simulink model "mfordmodel_v1"  (R2023a)
settings: Solver=ode45  StartTime=0.0  StopTime=10.0  RelTol=1e-3  EnableMultiTasking=on
undefined symbols (not defined in the file): ABV_RATIO_SW, AC_OFF_DLY, ACLOD, AUTO_TRNS_SW, BRAKE_DNDT_X, BZZRPM, BZZRPM_ALT, BZZTM, BZZTM_ALT, CMD_LITOFF, CMD_STABLE, CO_ST_ECT__A, COOL_BASE, DAS_BKDLY_A, DAS_CNT, DAS_CTDLY, DAS_LC_SW__A, DASCLP_5INH, DASCTL, DASMHYST, DASMPH, DEBYCP, DES_BASE, DPNEU_MUL, DSDRPM_DN_TC, DSDRPM_OFF, DSDRPM_UP_TC, EDF_DELAY, EDFHP, ETC_CL_TP, ETC_HP, GR_CM_CREEP, HCAM_ACT_CLP, HEDFHP, HEDFRPM, HICAM_PS, IAC_CAL_SW, IAC_ER_TM1, IAC_ER_TM2, IAC_ER_TM4, IAC_HI_LIM__A, IAC_ISFL_OBD, IAC_KAM_SW, IAC_LO_LIM__A, IAC_MON_TM, IAC_OT_REQ, IAC_RUN_TM, IAC_TP_OBD, IAC_TR_DAS, IAC_TST_DC, ID_DAS__A, ID_NOVS__A, IDVS_CH__A, IDVS_SL__A, IPSI_SW, IPSIDLY, IS_DRBASE__A, IS_DRBASE_A__A, IS_NUBASE__A, IS_NUBASE_A__A ... (+35)
libraries: simulink x2
(part 9 of 12)

== system mfordmodel_v1/iac_v04_001_001/normal_mode/iscflg_module/dashpot/TIMER/Time Calculator ==
  note: Calculates timer value.
      | Activated only when
      | counting up or down.
  note: Calculates time
      | between cycles.
      | Activated every cycle.
  note: Resets timer
      | to 'reset_value'
  note: Increment, hold,
      | or decrement
  note: Timer Control calls the counters 'delta_time' and 'timer_calculation'
      | after using the flags 'increment_flag' and 'decrement_flag'
      | to determine the direction of the timer.
  note: timer14/TIMER/Time Calculator
  count_direction : Inport
  reset_val : Inport  Port=2
  do_delta_time : Inport  Port=3
  do_timer : Inport  Port=4
  reset_value : Inport  Port=5
  From : From
  Goto : Goto
  delta_time : Subsystem  TreatAsAtomicUnit=on
  timer_calculation : Subsystem  TreatAsAtomicUnit=on
  timer : Outport
  wires:
  reset_value/1 -> timer_calculation/1(reset_value)  "reset_value"
  reset_val/1 -> timer_calculation/2(reset_flag)  "reset_flag"
  do_timer/1 -> timer_calculation/Trigger  "do_timer"
  From/1 -> timer_calculation/3(delta_time)  "delta_time"
  timer_calculation/1(timer) -> timer/1  "timer"
  count_direction/1 -> delta_time/1(count_direction)  "count_direction"
  delta_time/1(delta_time) -> Goto/1  "delta_time"
  do_delta_time/1 -> delta_time/Trigger  "do_delta_time"

== system mfordmodel_v1/iac_v04_001_001/normal_mode/iscflg_module/dashpot/daspot_calc/ROLAV_TC_in_DT_in ==
  note: Using the first two terms of the series expansion:
      |
      |                     x                     x2
      |                                e   =  1  +  x  +  --  + ......
      |                                           2!
      |
      |       Simplifying, the exponential "f" becomes:
      |
      |                  - (FK_TMR/TC)              1
      |           f  =  1  -  e                    =  1  -  -------------  =  . . .
      |                                                    (FK_TMR/TC)
      |                           e
      |
      |                              1                      1
      |          f  =  1  -  ---------------------------------  =    ------------------- .
      |                                  1 + (FK_TMR / TC)       1 + (TC / FK_TMR)
  note: - (FK_TMR/TC)
      |                                    f  =  1  -  e
      |
      |       Where "f" is called the filter constant in the difference equation:
      |
      |                    new_average = f * new_value + (1 - f) * old_average
  note: new_average = [ (sample_interval)/(sample_interval + time_constant) ] * (new_value - old_ave) + old_ave
  new_value : Inport
  Tau : Inport  Port=2
  old_ave : Inport  Port=3
  delta_time : Inport  Port=4
  Elementary Math : Math  Operator=reciprocal  SignedPower=on
  Product : Product  Inputs=3  InputSameDT=on  RndMeth=Zero  SaturateOnIntegerOverflow=on  OutDataTypeStr=Inherit: Same as first input
  Sum : Sum  Inputs=-+  InputSameDT=on  SaturateOnIntegerOverflow=on  OutDataTypeStr=Inherit: Same as first input
  Sum1 : Sum  InputSameDT=on  SaturateOnIntegerOverflow=on  OutDataTypeStr=Inherit: Same as first input
  Sum2 : Sum  InputSameDT=on  SaturateOnIntegerOverflow=on  OutDataTypeStr=Inherit: Same as first input
  new_ave : Outport
  wires:
  delta_time/1 -> Product/2, Sum1/1
  Tau/1 -> Sum1/2
  Sum2/1 -> new_ave/1
  old_ave/1 -> Sum2/1, Sum/1
  Product/1 -> Sum2/2
  Sum/1 -> Product/1
  Elementary Math/1 -> Product/3
  Sum1/1 -> Elementary Math/1
  new_value/1 -> Sum/2

== system mfordmodel_v1/iac_v04_001_001/normal_mode/iscflg_module/dashpot/daspot_calc/lookup_2d ==
  In1 : Inport
  Look-Up Table1 : Lookup  InputValues=calfunc.X  Table=calfunc.Y
  Saturation1 : Saturate  UpperLimit=max_x  LowerLimit=min_x
  Out1 : Outport
  wires:
  In1/1 -> Saturation1/1
  Saturation1/1 -> Look-Up Table1/1
  Look-Up Table1/1 -> Out1/1

== system mfordmodel_v1/iac_v04_001_001/normal_mode/iscflg_module/dashpot/daspot_calc/lookup_2d2 ==
  In1 : Inport
  Look-Up Table1 : Lookup  InputValues=calfunc.X  Table=calfunc.Y
  Saturation1 : Saturate  UpperLimit=max_x  LowerLimit=min_x
  Out1 : Outport
  wires:
  In1/1 -> Saturation1/1
  Saturation1/1 -> Look-Up Table1/1
  Look-Up Table1/1 -> Out1/1

== system mfordmodel_v1/iac_v04_001_001/normal_mode/iscflg_module/dashpot/function_calcs/lookup_2d ==
  In1 : Inport
  Look-Up Table1 : Lookup  InputValues=calfunc.X  Table=calfunc.Y
  Saturation1 : Saturate  UpperLimit=max_x  LowerLimit=min_x
  Out1 : Outport
  wires:
  In1/1 -> Saturation1/1
  Saturation1/1 -> Look-Up Table1/1
  Look-Up Table1/1 -> Out1/1

== system mfordmodel_v1/iac_v04_001_001/normal_mode/iscflg_module/dashpot/function_calcs/lookup_2d1 ==
  In1 : Inport
  Look-Up Table1 : Lookup  InputValues=calfunc.X  Table=calfunc.Y
  Saturation1 : Saturate  UpperLimit=max_x  LowerLimit=min_x
  Out1 : Outport
  wires:
  In1/1 -> Saturation1/1
  Saturation1/1 -> Look-Up Table1/1
  Look-Up Table1/1 -> Out1/1

== system mfordmodel_v1/iac_v04_001_001/normal_mode/iscflg_module/dashpot/function_calcs/lookup_2d2 ==
  In1 : Inport
  Look-Up Table1 : Lookup  InputValues=calfunc.X  Table=calfunc.Y
  Saturation1 : Saturate  UpperLimit=max_x  LowerLimit=min_x
  Out1 : Outport
  wires:
  In1/1 -> Saturation1/1
  Saturation1/1 -> Look-Up Table1/1
  Look-Up Table1/1 -> Out1/1

== system mfordmodel_v1/iac_v04_001_001/normal_mode/iscflg_module/dashpot/function_calcs/lookup_2d3 ==
  In1 : Inport
  Look-Up Table1 : Lookup  InputValues=calfunc.X  Table=calfunc.Y
  Saturation1 : Saturate  UpperLimit=max_x  LowerLimit=min_x
  Out1 : Outport
  wires:
  In1/1 -> Saturation1/1
  Saturation1/1 -> Look-Up Table1/1
  Look-Up Table1/1 -> Out1/1

== system mfordmodel_v1/iac_v04_001_001/normal_mode/iscflg_module/dashpot/function_calcs/lookup_2d4 ==
  In1 : Inport
  Look-Up Table1 : Lookup  InputValues=calfunc.X  Table=calfunc.Y
  Saturation1 : Saturate  UpperLimit=max_x  LowerLimit=min_x
  Out1 : Outport
  wires:
  In1/1 -> Saturation1/1
  Saturation1/1 -> Look-Up Table1/1
  Look-Up Table1/1 -> Out1/1

== system mfordmodel_v1/iac_v04_001_001/normal_mode/iscflg_module/dashpot/function_calcs/lookup_2d5 ==
  In1 : Inport
  Look-Up Table1 : Lookup  InputValues=calfunc.X  Table=calfunc.Y
  Saturation1 : Saturate  UpperLimit=max_x  LowerLimit=min_x
  Out1 : Outport
  wires:
  In1/1 -> Saturation1/1
  Saturation1/1 -> Look-Up Table1/1
  Look-Up Table1/1 -> Out1/1

== system mfordmodel_v1/iac_v04_001_001/normal_mode/iscflg_module/dashpot/function_calcs/lookup_2d6 ==
  In1 : Inport
  Look-Up Table1 : Lookup  InputValues=calfunc.X  Table=calfunc.Y
  Saturation1 : Saturate  UpperLimit=max_x  LowerLimit=min_x
  Out1 : Outport
  wires:
  In1/1 -> Saturation1/1
  Saturation1/1 -> Look-Up Table1/1
  Look-Up Table1/1 -> Out1/1

== system mfordmodel_v1/iac_v04_001_001/normal_mode/iscflg_module/dashpot/function_calcs/lookup_2d7 ==
  In1 : Inport
  Look-Up Table1 : Lookup  InputValues=calfunc.X  Table=calfunc.Y
  Saturation1 : Saturate  UpperLimit=max_x  LowerLimit=min_x
  Out1 : Outport
  wires:
  In1/1 -> Saturation1/1
  Saturation1/1 -> Look-Up Table1/1
  Look-Up Table1/1 -> Out1/1

== system mfordmodel_v1/iac_v04_001_001/normal_mode/iscflg_module/idle_drive_rpm_controller/idle_ppm_calc/ 1 ==
  In1 : Inport
  Look-Up Table1 : Lookup  InputValues=calfunc.X  Table=calfunc.Y
  Saturation1 : Saturate  UpperLimit=max_x  LowerLimit=min_x
  Out1 : Outport
  wires:
  In1/1 -> Saturation1/1
  Saturation1/1 -> Look-Up Table1/1
  Look-Up Table1/1 -> Out1/1

== system mfordmodel_v1/iac_v04_001_001/normal_mode/iscflg_module/idle_drive_rpm_controller/idle_ppm_calc/CONSTANT7 ==
  Constant : Constant  Value=const
  Out : Outport
  wires:
  Constant/1 -> Out/1

== system mfordmodel_v1/iac_v04_001_001/normal_mode/iscflg_module/idle_drive_rpm_controller/idle_ppm_calc/CONSTANT8 ==
  Constant : Constant  Value=const
  Out : Outport
  wires:
  Constant/1 -> Out/1

== system mfordmodel_v1/iac_v04_001_001/normal_mode/iscflg_module/idle_drive_rpm_controller/idle_ppm_calc/CONSTANT9 ==
  Constant : Constant  Value=const
  Out : Outport
  wires:
  Constant/1 -> Out/1

== system mfordmodel_v1/iac_v04_001_001/normal_mode/iscflg_module/idle_drive_rpm_controller/idle_ppm_calc/VAR_SATURATION1 ==
  note: IF INPUT <= MIN THEN SWITCH MIN ON
  note: IF INPUT >= MAX THEN SWITHMAX ON
  MAX : Inport
  INPUT : Inport  Port=2
  MIN : Inport  Port=3
  From : From
  From1 : From
  Goto : Goto
  Logical Operator : Logic  Operator=OR
  Relational Operator : RelationalOperator
  Relational Operator1 : RelationalOperator  Operator=<=
  Switch : Switch  Threshold=0.5
  Switch2 : Switch  Threshold=0.5
  SwitchMAX : Switch  Threshold=0.5
  OUTPUT : Outport
  LIMIT_FLAG : Outport  Port=2
  wires:
  MIN/1 -> Switch/1, Relational Operator1/2
  Switch/1 -> Switch2/3
  From1/1 -> SwitchMAX/3
  From/1 -> Switch/3
  INPUT/1 -> Goto/1, Relational Operator1/1, Relational Operator/1
  Switch2/1 -> OUTPUT/1
  SwitchMAX/1 -> Switch2/1
  MAX/1 -> SwitchMAX/1, Relational Operator/2
  Relational Operator/1 -> SwitchMAX/2, Switch2/2, Logical Operator/1
  Relational Operator1/1 -> Switch/2, Logical Operator/2
  Logical Operator/1 -> LIMIT_FLAG/1

== system mfordmodel_v1/iac_v04_001_001/normal_mode/iscflg_module/idle_drive_rpm_controller/idle_ppm_calc/VAR_SATURATION2 ==
  note: IF INPUT <= MIN THEN SWITCH MIN ON
  note: IF INPUT >= MAX THEN SWITHMAX ON
  MAX : Inport
  INPUT : Inport  Port=2
  MIN : Inport  Port=3
  From : From
  From1 : From
  Goto : Goto
  Logical Operator : Logic  Operator=OR
  Relational Operator : RelationalOperator
  Relational Operator1 : RelationalOperator  Operator=<=
  Switch : Switch  Threshold=0.5
  Switch2 : Switch  Threshold=0.5
  SwitchMAX : Switch  Threshold=0.5
  OUTPUT : Outport
  LIMIT_FLAG : Outport  Port=2
  wires:
  MIN/1 -> Switch/1, Relational Operator1/2
  Switch/1 -> Switch2/3
  From1/1 -> SwitchMAX/3
  From/1 -> Switch/3
  INPUT/1 -> Goto/1, Relational Operator1/1, Relational Operator/1
  Switch2/1 -> OUTPUT/1
  SwitchMAX/1 -> Switch2/1
  MAX/1 -> SwitchMAX/1, Relational Operator/2
  Relational Operator/1 -> SwitchMAX/2, Switch2/2, Logical Operator/1
  Relational Operator1/1 -> Switch/2, Logical Operator/2
  Logical Operator/1 -> LIMIT_FLAG/1

== system mfordmodel_v1/iac_v04_001_001/normal_mode/iscflg_module/idle_drive_rpm_controller/idnerr_fil_calc/CONSTANT1 ==
  Constant : Constant  Value=const
  Out : Outport
  wires:
  Constant/1 -> Out/1

== system mfordmodel_v1/iac_v04_001_001/normal_mode/iscflg_module/idle_drive_rpm_controller/idnerr_fil_calc/ROLAV_TC_DT_in1 ==
  note: Using the first two terms of the series expansion:
      |
      |                     x                     x2
      |                                e   =  1  +  x  +  --  + ......
      |                                           2!
      |
      |       Simplifying, the exponential "f" becomes:
      |
      |                  - (FK_TMR/TC)              1
      |           f  =  1  -  e                    =  1  -  -------------  =  . . .
      |                                                    (FK_TMR/TC)
      |                           e
      |
      |                              1                      1
      |          f  =  1  -  ---------------------------------  =    ------------------- .
      |                                  1 + (FK_TMR / TC)       1 + (TC / FK_TMR)
  note: - (FK_TMR/TC)
      |                                    f  =  1  -  e
      |
      |       Where "f" is called the filter constant in the difference equation:
      |
      |                    new_average = f * new_value + (1 - f) * old_average
  note: new_average = [ (sample_interval)/(sample_interval + time_constant) ] * (new_value - old_ave) + old_ave
  new_value : Inport
  old_ave : Inport  Port=2
  delta_time : Inport  Port=3
  Elementary Math : Math  Operator=reciprocal  SignedPower=on
  Product : Product  Inputs=3  InputSameDT=on  RndMeth=Zero  SaturateOnIntegerOverflow=on  OutDataTypeStr=Inherit: Same as first input
  Sum : Sum  Inputs=-+  InputSameDT=on  SaturateOnIntegerOverflow=on  OutDataTypeStr=Inherit: Same as first input
  Sum1 : Sum  InputSameDT=on  SaturateOnIntegerOverflow=on  OutDataTypeStr=Inherit: Same as first input
  Sum2 : Sum  InputSameDT=on  SaturateOnIntegerOverflow=on  OutDataTypeStr=Inherit: Same as first input
  Time Constant : Constant  Value=tc
  new_ave : Outport
  wires:
  Time Constant/1 -> Sum1/2
  Sum2/1 -> new_ave/1
  old_ave/1 -> Sum2/1, Sum/1
  Product/1 -> Sum2/2
  Sum/1 -> Product/1
  Elementary Math/1 -> Product/3
  Sum1/1 -> Elementary Math/1
  new_value/1 -> Sum/2
  delta_time/1 -> Product/2, Sum1/1

== system mfordmodel_v1/iac_v04_001_001/normal_mode/iscflg_module/idle_rpm_controller/fn852a_calc/FN852A ==
  In1 : Inport
  Look-Up Table1 : Lookup  InputValues=calfunc.X  Table=calfunc.Y
  Saturation1 : Saturate  UpperLimit=max_x  LowerLimit=min_x
  Out1 : Outport
  wires:
  In1/1 -> Saturation1/1
  Saturation1/1 -> Look-Up Table1/1
  Look-Up Table1/1 -> Out1/1

== system mfordmodel_v1/iac_v04_001_001/normal_mode/iscflg_module/idle_rpm_controller/idle_ppm_calc/FN851A ==
  In1 : Inport
  Look-Up Table1 : Lookup  InputValues=calfunc.X  Table=calfunc.Y
  Saturation1 : Saturate  UpperLimit=max_x  LowerLimit=min_x
  Out1 : Outport
  wires:
  In1/1 -> Saturation1/1
  Saturation1/1 -> Look-Up Table1/1
  Look-Up Table1/1 -> Out1/1

== system mfordmodel_v1/iac_v04_001_001/normal_mode/iscflg_module/idle_rpm_controller/idle_ppm_calc/PID_DELTA ==
  Constant : Constant  Value=const
  Out : Outport
  wires:
  Constant/1 -> Out/1

== system mfordmodel_v1/iac_v04_001_001/normal_mode/iscflg_module/idle_rpm_controller/idle_ppm_calc/ROLAV_TC_in_DT_in ==
  note: Using the first two terms of the series expansion:
      |
      |                     x                     x2
      |                                e   =  1  +  x  +  --  + ......
      |                                           2!
      |
      |       Simplifying, the exponential "f" becomes:
      |
      |                  - (FK_TMR/TC)              1
      |           f  =  1  -  e                    =  1  -  -------------  =  . . .
      |                                                    (FK_TMR/TC)
      |                           e
      |
      |                              1                      1
      |          f  =  1  -  ---------------------------------  =    ------------------- .
      |                                  1 + (FK_TMR / TC)       1 + (TC / FK_TMR)
  note: - (FK_TMR/TC)
      |                                    f  =  1  -  e
      |
      |       Where "f" is called the filter constant in the difference equation:
      |
      |                    new_average = f * new_value + (1 - f) * old_average
  note: new_average = [ (sample_interval)/(sample_interval + time_constant) ] * (new_value - old_ave) + old_ave
  new_value : Inport
  Tau : Inport  Port=2
  old_ave : Inport  Port=3
  delta_time : Inport  Port=4
  Elementary Math : Math  Operator=reciprocal  SignedPower=on
  Product : Product  Inputs=3  InputSameDT=on  RndMeth=Zero  SaturateOnIntegerOverflow=on  OutDataTypeStr=Inherit: Same as first input
  Sum : Sum  Inputs=-+  InputSameDT=on  SaturateOnIntegerOverflow=on  OutDataTypeStr=Inherit: Same as first input
  Sum1 : Sum  InputSameDT=on  SaturateOnIntegerOverflow=on  OutDataTypeStr=Inherit: Same as first input
  Sum2 : Sum  InputSameDT=on  SaturateOnIntegerOverflow=on  OutDataTypeStr=Inherit: Same as first input
  new_ave : Outport
  wires:
  delta_time/1 -> Product/2, Sum1/1
  Tau/1 -> Sum1/2
  Sum2/1 -> new_ave/1
  old_ave/1 -> Sum2/1, Sum/1
  Product/1 -> Sum2/2
  Sum/1 -> Product/1
  Elementary Math/1 -> Product/3
  Sum1/1 -> Elementary Math/1
  new_value/1 -> Sum/2

== system mfordmodel_v1/iac_v04_001_001/normal_mode/iscflg_module/idle_rpm_controller/idle_ppm_calc/ROLAV_TC_in_DT_in1 ==
  note: Using the first two terms of the series expansion:
      |
      |                     x                     x2
      |                                e   =  1  +  x  +  --  + ......
      |                                           2!
      |
      |       Simplifying, the exponential "f" becomes:
      |
      |                  - (FK_TMR/TC)              1
      |           f  =  1  -  e                    =  1  -  -------------  =  . . .
      |                                                    (FK_TMR/TC)
      |                           e
      |
      |                              1                      1
      |          f  =  1  -  ---------------------------------  =    ------------------- .
      |                                  1 + (FK_TMR / TC)       1 + (TC / FK_TMR)
  note: - (FK_TMR/TC)
      |                                    f  =  1  -  e
      |
      |       Where "f" is called the filter constant in the difference equation:
      |
      |                    new_average = f * new_value + (1 - f) * old_average
  note: new_average = [ (sample_interval)/(sample_interval + time_constant) ] * (new_value - old_ave) + old_ave
  new_value : Inport
  Tau : Inport  Port=2
  old_ave : Inport  Port=3
  delta_time : Inport  Port=4
  Elementary Math : Math  Operator=reciprocal  SignedPower=on
  Product : Product  Inputs=3  InputSameDT=on  RndMeth=Zero  SaturateOnIntegerOverflow=on  OutDataTypeStr=Inherit: Same as first input
  Sum : Sum  Inputs=-+  InputSameDT=on  SaturateOnIntegerOverflow=on  OutDataTypeStr=Inherit: Same as first input
  Sum1 : Sum  InputSameDT=on  SaturateOnIntegerOverflow=on  OutDataTypeStr=Inherit: Same as first input
  Sum2 : Sum  InputSameDT=on  SaturateOnIntegerOverflow=on  OutDataTypeStr=Inherit: Same as first input
  new_ave : Outport
  wires:
  delta_time/1 -> Product/2, Sum1/1
  Tau/1 -> Sum1/2
  Sum2/1 -> new_ave/1
  old_ave/1 -> Sum2/1, Sum/1
  Product/1 -> Sum2/2
  Sum/1 -> Product/1
  Elementary Math/1 -> Product/3
  Sum1/1 -> Elementary Math/1
  new_value/1 -> Sum/2

== system mfordmodel_v1/iac_v04_001_001/normal_mode/iscflg_module/idle_rpm_controller/idle_ppm_calc/TCBPA_DER ==
  Constant : Constant  Value=const
  Out : Outport
  wires:
  Constant/1 -> Out/1

== system mfordmodel_v1/iac_v04_001_001/normal_mode/iscflg_module/idle_rpm_controller/idle_ppm_calc/TCPRO_GT ==
  Constant : Constant  Value=const
  Out : Outport
  wires:
  Constant/1 -> Out/1

== system mfordmodel_v1/iac_v04_001_001/normal_mode/iscflg_module/idle_rpm_controller/idle_ppm_calc/TCPRO_LT ==
  Constant : Constant  Value=const
  Out : Outport
  wires:
  Constant/1 -> Out/1

== system mfordmodel_v1/iac_v04_001_001/normal_mode/iscflg_module/idle_rpm_controller/iscpsi_calc/TC_OVER ==
  Constant : Constant  Value=const
  Out : Outport
  wires:
  Constant/1 -> Out/1

== system mfordmodel_v1/iac_v04_001_001/normal_mode/iscflg_module/idle_rpm_controller/iscpsi_calc/TC_UNDER ==
  Constant : Constant  Value=const
  Out : Outport
  wires:
  Constant/1 -> Out/1

== system mfordmodel_v1/iac_v04_001_001/normal_mode/iscflg_module/idle_rpm_controller/rpmerr_calc/ROLAV_TC_DT_in ==
  note: Using the first two terms of the series expansion:
      |
      |                     x                     x2
      |                                e   =  1  +  x  +  --  + ......
      |                                           2!
      |
      |       Simplifying, the exponential "f" becomes:
      |
      |                  - (FK_TMR/TC)              1
      |           f  =  1  -  e                    =  1  -  -------------  =  . . .
      |                                                    (FK_TMR/TC)
      |                           e
      |
      |                              1                      1
      |          f  =  1  -  ---------------------------------  =    ------------------- .
      |                                  1 + (FK_TMR / TC)       1 + (TC / FK_TMR)
  note: - (FK_TMR/TC)
      |                                    f  =  1  -  e
      |
      |       Where "f" is called the filter constant in the difference equation:
      |
      |                    new_average = f * new_value + (1 - f) * old_average
  note: new_average = [ (sample_interval)/(sample_interval + time_constant) ] * (new_value - old_ave) + old_ave
  new_value : Inport
  old_ave : Inport  Port=2
  delta_time : Inport  Port=3
  Elementary Math : Math  Operator=reciprocal  SignedPower=on
  Product : Product  Inputs=3  InputSameDT=on  RndMeth=Zero  SaturateOnIntegerOverflow=on  OutDataTypeStr=Inherit: Same as first input
  Sum : Sum  Inputs=-+  InputSameDT=on  SaturateOnIntegerOverflow=on  OutDataTypeStr=Inherit: Same as first input
  Sum1 : Sum  InputSameDT=on  SaturateOnIntegerOverflow=on  OutDataTypeStr=Inherit: Same as first input
  Sum2 : Sum  InputSameDT=on  SaturateOnIntegerOverflow=on  OutDataTypeStr=Inherit: Same as first input
  Time Constant : Constant  Value=tc
  new_ave : Outport
  wires:
  Time Constant/1 -> Sum1/2
  Sum2/1 -> new_ave/1
  old_ave/1 -> Sum2/1, Sum/1
  Product/1 -> Sum2/2
  Sum/1 -> Product/1
  Elementary Math/1 -> Product/3
  Sum1/1 -> Elementary Math/1
  new_value/1 -> Sum/2
  delta_time/1 -> Product/2, Sum1/1

== system mfordmodel_v1/iac_v04_001_001/normal_mode/iscflg_module/iscflg_modes/1/Time Calculator ==
  note: Calculates timer value.
      | Activated only when
      | counting up or down.
  note: Calculates time
      | between cycles.
      | Activated every cycle.
  note: Resets timer
      | to 'reset_value'
  note: Increment, hold,
      | or decrement
  note: Timer Control calls the counters 'delta_time' and 'timer_calculation'
      | after using the flags 'increment_flag' and 'decrement_flag'
      | to determine the direction of the timer.
  note: timer14/TIMER/Time Calculator
  count_direction : Inport
  reset_val : Inport  Port=2
  do_delta_time : Inport  Port=3
  do_timer : Inport  Port=4
  reset_value : Inport  Port=5
  From : From
  Goto : Goto
  delta_time : Subsystem  TreatAsAtomicUnit=on
  timer_calculation : Subsystem  TreatAsAtomicUnit=on
  timer : Outport
  wires:
  reset_value/1 -> timer_calculation/1(reset_value)  "reset_value"
  reset_val/1 -> timer_calculation/2(reset_flag)  "reset_flag"
  do_timer/1 -> timer_calculation/Trigger  "do_timer"
  From/1 -> timer_calculation/3(delta_time)  "delta_time"
  timer_calculation/1(timer) -> timer/1  "timer"
  count_direction/1 -> delta_time/1(count_direction)  "count_direction"
  delta_time/1(delta_time) -> Goto/1  "delta_time"
  do_delta_time/1 -> delta_time/Trigger  "do_delta_time"

== system mfordmodel_v1/iac_v04_001_001/normal_mode/iscflg_module/iscflg_modes/2/Time Calculator ==
  note: Calculates timer value.
      | Activated only when
      | counting up or down.
  note: Calculates time
      | between cycles.
      | Activated every cycle.
  note: Resets timer
      | to 'reset_value'
  note: Increment, hold,
      | or decrement
  note: Timer Control calls the counters 'delta_time' and 'timer_calculation'
      | after using the flags 'increment_flag' and 'decrement_flag'
      | to determine the direction of the timer.
  note: timer14/TIMER/Time Calculator
  count_direction : Inport
  reset_val : Inport  Port=2
  do_delta_time : Inport  Port=3
  do_timer : Inport  Port=4
  reset_value : Inport  Port=5
  From : From
  Goto : Goto
  delta_time : Subsystem  TreatAsAtomicUnit=on
  timer_calculation : Subsystem  TreatAsAtomicUnit=on
  timer : Outport
  wires:
  reset_value/1 -> timer_calculation/1(reset_value)  "reset_value"
  reset_val/1 -> timer_calculation/2(reset_flag)  "reset_flag"
  do_timer/1 -> timer_calculation/Trigger  "do_timer"
  From/1 -> timer_calculation/3(delta_time)  "delta_time"
  timer_calculation/1(timer) -> timer/1  "timer"
  count_direction/1 -> delta_time/1(count_direction)  "count_direction"
  delta_time/1(delta_time) -> Goto/1  "delta_time"
  do_delta_time/1 -> delta_time/Trigger  "do_delta_time"

== system mfordmodel_v1/iac_v04_001_001/normal_mode/iscflg_module/preposition/idle_ppm_calc/CONSTANT ==
  Constant : Constant  Value=const
  Out : Outport
  wires:
  Constant/1 -> Out/1

== system mfordmodel_v1/iac_v04_001_001/normal_mode/iscflg_module/preposition/idle_ppm_calc/CONSTANT1 ==
  Constant : Constant  Value=const
  Out : Outport
  wires:
  Constant/1 -> Out/1

== system mfordmodel_v1/iac_v04_001_001/normal_mode/iscflg_module/preposition/idle_ppm_calc/CONSTANT2 ==
  Constant : Constant  Value=const
  Out : Outport
  wires:
  Constant/1 -> Out/1

== system mfordmodel_v1/iac_v04_001_001/normal_mode/iscflg_module/preposition/idle_ppm_calc/FN814 ==
  In1 : Inport
  Look-Up Table1 : Lookup  InputValues=calfunc.X  Table=calfunc.Y
  Saturation1 : Saturate  UpperLimit=max_x  LowerLimit=min_x
  Out1 : Outport
  wires:
  In1/1 -> Saturation1/1
  Saturation1/1 -> Look-Up Table1/1
  Look-Up Table1/1 -> Out1/1

== system mfordmodel_v1/iac_v04_001_001/normal_mode/iscflg_module/preposition/idle_ppm_calc/FN830__A ==
  In1 : Inport
  Look-Up Table1 : Lookup  InputValues=calfunc.X  Table=calfunc.Y
  Saturation1 : Saturate  UpperLimit=max_x  LowerLimit=min_x
  Out1 : Outport
  wires:
  In1/1 -> Saturation1/1
  Saturation1/1 -> Look-Up Table1/1
  Look-Up Table1/1 -> Out1/1

== system mfordmodel_v1/iac_v04_001_001/normal_mode/iscflg_module/preposition/idle_ppm_calc/FN882A1 ==
  In1 : Inport
  Look-Up Table1 : Lookup  InputValues=calfunc.X  Table=calfunc.Y
  Saturation1 : Saturate  UpperLimit=max_x  LowerLimit=min_x
  Out1 : Outport
  wires:
  In1/1 -> Saturation1/1
  Saturation1/1 -> Look-Up Table1/1
  Look-Up Table1/1 -> Out1/1

== system mfordmodel_v1/iac_v04_001_001/normal_mode/iscflg_module/preposition/idle_ppm_calc/FN891 ==
  In1 : Inport
  Look-Up Table1 : Lookup  InputValues=calfunc.X  Table=calfunc.Y
  Saturation1 : Saturate  UpperLimit=max_x  LowerLimit=min_x
  Out1 : Outport
  wires:
  In1/1 -> Saturation1/1
  Saturation1/1 -> Look-Up Table1/1
  Look-Up Table1/1 -> Out1/1

== system mfordmodel_v1/iac_v04_001_001/iac_executive/fault_code_setting/TIMER_DT_in/Time Calculator/timer_calculation/VAR SATURATION ==
  note: IF INPUT >= MAX THEN SWITHMAX ON
  note: IF INPUT <= MIN THEN SWITCH MIN ON
  MAX : Inport
  INPUT : Inport  Port=2
  MIN : Inport  Port=3
  From : From
  From1 : From
  Goto : Goto
  Logical Operator : Logic  Operator=OR
  Relational Operator : RelationalOperator
  Relational Operator1 : RelationalOperator  Operator=<=
  Switch : Switch  Threshold=0.5
  Switch2 : Switch  Threshold=0.5
  SwitchMAX : Switch  Threshold=0.5
  OUTPUT : Outport
  LIMIT_FLAG : Outport  Port=2
  wires:
  Logical Operator/1 -> LIMIT_FLAG/1
  Relational Operator1/1 -> Logical Operator/2, Switch/2
  Relational Operator/1 -> Logical Operator/1, Switch2/2, SwitchMAX/2
  MAX/1 -> Relational Operator/2, SwitchMAX/1
  SwitchMAX/1 -> Switch2/1
  Switch2/1 -> OUTPUT/1
  INPUT/1 -> Relational Operator/1, Relational Operator1/1, Goto/1
  From/1 -> Switch/3
  From1/1 -> SwitchMAX/3
  Switch/1 -> Switch2/3
  MIN/1 -> Relational Operator1/2, Switch/1

== system mfordmodel_v1/iac_v04_001_001/iac_executive/misc_calcs/TIMER_DT_in/Time Calculator/timer_calculation/VAR SATURATION ==
  note: IF INPUT >= MAX THEN SWITHMAX ON
  note: IF INPUT <= MIN THEN SWITCH MIN ON
  MAX : Inport
  INPUT : Inport  Port=2
  MIN : Inport  Port=3
  From : From
  From1 : From
  Goto : Goto
  Logical Operator : Logic  Operator=OR
  Relational Operator : RelationalOperator
  Relational Operator1 : RelationalOperator  Operator=<=
  Switch : Switch  Threshold=0.5
  Switch2 : Switch  Threshold=0.5
  SwitchMAX : Switch  Threshold=0.5
  OUTPUT : Outport
  LIMIT_FLAG : Outport  Port=2
  wires:
  Logical Operator/1 -> LIMIT_FLAG/1
  Relational Operator1/1 -> Logical Operator/2, Switch/2
  Relational Operator/1 -> Logical Operator/1, Switch2/2, SwitchMAX/2
  MAX/1 -> Relational Operator/2, SwitchMAX/1
  SwitchMAX/1 -> Switch2/1
  Switch2/1 -> OUTPUT/1
  INPUT/1 -> Relational Operator/1, Relational Operator1/1, Goto/1
  From/1 -> Switch/3
  From1/1 -> SwitchMAX/3
  Switch/1 -> Switch2/3
  MIN/1 -> Relational Operator1/2, Switch/1

== system mfordmodel_v1/iac_v04_001_001/iac_executive/runup_flag_timer/TIMER_DT_in/Time Calculator/timer_calculation/VAR SATURATION ==
  note: IF INPUT >= MAX THEN SWITHMAX ON
  note: IF INPUT <= MIN THEN SWITCH MIN ON
  MAX : Inport
  INPUT : Inport  Port=2
  MIN : Inport  Port=3
  From : From
  From1 : From
  Goto : Goto
  Logical Operator : Logic  Operator=OR
  Relational Operator : RelationalOperator
  Relational Operator1 : RelationalOperator  Operator=<=
  Switch : Switch  Threshold=0.5
  Switch2 : Switch  Threshold=0.5
  SwitchMAX : Switch  Threshold=0.5
  OUTPUT : Outport
  LIMIT_FLAG : Outport  Port=2
  wires:
  Logical Operator/1 -> LIMIT_FLAG/1
  Relational Operator1/1 -> Logical Operator/2, Switch/2
  Relational Operator/1 -> Logical Operator/1, Switch2/2, SwitchMAX/2
  MAX/1 -> Relational Operator/2, SwitchMAX/1
  SwitchMAX/1 -> Switch2/1
  Switch2/1 -> OUTPUT/1
  INPUT/1 -> Relational Operator/1, Relational Operator1/1, Goto/1
  From/1 -> Switch/3
  From1/1 -> SwitchMAX/3
  Switch/1 -> Switch2/3
  MIN/1 -> Relational Operator1/2, Switch/1

== system mfordmodel_v1/iac_v04_001_001/normal_mode/activate_feedforward/ac_ppm_tmr/Time Calculator/timer_calculation/VAR SATURATION ==
  note: IF INPUT >= MAX THEN SWITHMAX ON
  note: IF INPUT <= MIN THEN SWITCH MIN ON
  MAX : Inport
  INPUT : Inport  Port=2
  MIN : Inport  Port=3
  From : From
  From1 : From
  Goto : Goto
  Logical Operator : Logic  Operator=OR
  Relational Operator : RelationalOperator
  Relational Operator1 : RelationalOperator  Operator=<=
  Switch : Switch  Threshold=0.5
  Switch2 : Switch  Threshold=0.5
  SwitchMAX : Switch  Threshold=0.5
  OUTPUT : Outport
  LIMIT_FLAG : Outport  Port=2
  wires:
  Logical Operator/1 -> LIMIT_FLAG/1
  Relational Operator1/1 -> Logical Operator/2, Switch/2
  Relational Operator/1 -> Logical Operator/1, Switch2/2, SwitchMAX/2
  MAX/1 -> Relational Operator/2, SwitchMAX/1
  SwitchMAX/1 -> Switch2/1
  Switch2/1 -> OUTPUT/1
  INPUT/1 -> Relational Operator/1, Relational Operator1/1, Goto/1
  From/1 -> Switch/3
  From1/1 -> SwitchMAX/3
  Switch/1 -> Switch2/3
  MIN/1 -> Relational Operator1/2, Switch/1

== system mfordmodel_v1/iac_v04_001_001/normal_mode/activate_kam/iac_kam_tmr/Time Calculator/timer_calculation/VAR SATURATION ==
  note: IF INPUT >= MAX THEN SWITHMAX ON
  note: IF INPUT <= MIN THEN SWITCH MIN ON
  MAX : Inport
  INPUT : Inport  Port=2
  MIN : Inport  Port=3
  From : From
  From1 : From
  Goto : Goto
  Logical Operator : Logic  Operator=OR
  Relational Operator : RelationalOperator
  Relational Operator1 : RelationalOperator  Operator=<=
  Switch : Switch  Threshold=0.5
  Switch2 : Switch  Threshold=0.5
  SwitchMAX : Switch  Threshold=0.5
  OUTPUT : Outport
  LIMIT_FLAG : Outport  Port=2
  wires:
  Logical Operator/1 -> LIMIT_FLAG/1
  Relational Operator1/1 -> Logical Operator/2, Switch/2
  Relational Operator/1 -> Logical Operator/1, Switch2/2, SwitchMAX/2
  MAX/1 -> Relational Operator/2, SwitchMAX/1
  SwitchMAX/1 -> Switch2/1
  Switch2/1 -> OUTPUT/1
  INPUT/1 -> Relational Operator/1, Relational Operator1/1, Goto/1
  From/1 -> Switch/3
  From1/1 -> SwitchMAX/3
  Switch/1 -> Switch2/3
  MIN/1 -> Relational Operator1/2, Switch/1

== system mfordmodel_v1/iac_v04_001_001/normal_mode/activate_normal_mode/normal_mode_fault_codes/iac_er_tmr1/Time Calculator/delta_time ==
  note: timer14/TIMER/Time Calculator/delta_time
  note: Timer direction is represented by
      | the multiplier 'count_direction'
      | 'count_direction' can be either -1, 0, or 1.
  note: 'delta_time': the time interval
      | to be added to the timer for each cycle.
      | 'Gain' will adjust for second or millisecond timers.
  count_direction : Inport
  do_delta_time : TriggerPort  TriggerType=function-call  VariantControl=(inherit)
  Gain : Gain  Gain=unit_mul  SaturateOnIntegerOverflow=on  OutDataTypeStr=Inherit: Same as input  ParamDataTypeStr=Inherit: Same as input
  Product : Product  InputSameDT=on  RndMeth=Zero  SaturateOnIntegerOverflow=on  OutDataTypeStr=Inherit: Same as first input
  Realtime Digital Clock : DigitalClock  SampleTime=-1
  Sum : Sum  Inputs=+-  InputSameDT=on  SaturateOnIntegerOverflow=on  OutDataTypeStr=Inherit: Same as first input
  Unit Delay1 : UnitDelay  SampleTime=-1
  delta_time : Outport  InitialOutput=0
  wires:
  Realtime Digital Clock/1 -> Sum/1, Unit Delay1/1  "timer"
  Gain/1 -> Product/2
  Sum/1 -> Gain/1
  Unit Delay1/1 -> Sum/2
  Product/1 -> delta_time/1  "delta_time"
  count_direction/1 -> Product/1  "count_direction"

== system mfordmodel_v1/iac_v04_001_001/normal_mode/activate_normal_mode/normal_mode_fault_codes/iac_er_tmr1/Time Calculator/timer_calculation ==
  note: When 'reset_flag' is 1,
      |  'reset_value' is selected and
      | passed through the timer.
  note: 'init_value' provides the
      | initial value for the timer
  note: 'timer': cumulative
      | timer value
  note: 'Quantizer' switches the output
      |  to the appropriate resolution
      | based upon the top level
      |  dialog box selection.
  note: 'timer_calculation' takes the directional time increment 'delta_time'
      | and adds it to the previous timer value.  When the timer is reset,
      | all values are reset to 'reset_value'.
  reset_value : Inport
  reset_flag : Inport  Port=2
  delta_time : Inport  Port=3
  do_timer : TriggerPort  TriggerType=function-call  VariantControl=(inherit)
  Constant1 : Constant  Value=const_min
  Constant2 : Constant  Value=const_max
  Quantizer5 : Fcn  Expr=resolution*floor(u/resolution)
  Reset Switch : Switch  Threshold=0.5
  Sum : Sum  InputSameDT=on  SaturateOnIntegerOverflow=on  OutDataTypeStr=Inherit: Same as first input
  Terminator : Terminator
  Unit Delay : UnitDelay  InitialCondition=init_value  SampleTime=-1
  VAR SATURATION : Subsystem  mask(VARIABLE SATURATION){}
      mask help: This block will clip the input between the MIN and MAX values specified as inputs to the block. In addition a LIMIT_FLAG will be set to 1 if the input is currently being clipped.
      mask Display:
      | plot( [0.2 0.3 0.5 0.6], [0.2 0.2 0.8 0.8])
      | text(0.2, 0.05, 'min')
      | text(0.5, 0.95, 'max')
  lower bound = 0 : DeadZone  LowerValue=-inf  UpperValue=0.0
  timer : Outport  InitialOutput=0
  wires:
  Quantizer5/1 -> timer/1  "timer"
  VAR SATURATION/1(OUTPUT) -> Quantizer5/1, Unit Delay/1
  Sum/1 -> Reset Switch/3
  delta_time/1 -> Sum/1  "delta_time"
  reset_value/1 -> Reset Switch/1  "reset_value"
  reset_flag/1 -> Reset Switch/2  "reset_flag"
  Reset Switch/1 -> lower bound = 0/1
  Unit Delay/1 -> Sum/2  "previous  timer value"
  lower bound = 0/1 -> VAR SATURATION/2(INPUT)
  Constant1/1 -> VAR SATURATION/3(MIN)
  Constant2/1 -> VAR SATURATION/1(MAX)
  VAR SATURATION/2(LIMIT_FLAG) -> Terminator/1

== system mfordmodel_v1/iac_v04_001_001/normal_mode/activate_normal_mode/normal_mode_fault_codes/iac_er_tmr2/Time Calculator/delta_time ==
  note: timer14/TIMER/Time Calculator/delta_time
  note: Timer direction is represented by
      | the multiplier 'count_direction'
      | 'count_direction' can be either -1, 0, or 1.
  note: 'delta_time': the time interval
      | to be added to the timer for each cycle.
      | 'Gain' will adjust for second or millisecond timers.
  count_direction : Inport
  do_delta_time : TriggerPort  TriggerType=function-call  VariantControl=(inherit)
  Gain : Gain  Gain=unit_mul  SaturateOnIntegerOverflow=on  OutDataTypeStr=Inherit: Same as input  ParamDataTypeStr=Inherit: Same as input
  Product : Product  InputSameDT=on  RndMeth=Zero  SaturateOnIntegerOverflow=on  OutDataTypeStr=Inherit: Same as first input
  Realtime Digital Clock : DigitalClock  SampleTime=-1
  Sum : Sum  Inputs=+-  InputSameDT=on  SaturateOnIntegerOverflow=on  OutDataTypeStr=Inherit: Same as first input
  Unit Delay1 : UnitDelay  SampleTime=-1
  delta_time : Outport  InitialOutput=0
  wires:
  Realtime Digital Clock/1 -> Sum/1, Unit Delay1/1  "timer"
  Gain/1 -> Product/2
  Sum/1 -> Gain/1
  Unit Delay1/1 -> Sum/2
  Product/1 -> delta_time/1  "delta_time"
  count_direction/1 -> Product/1  "count_direction"

== system mfordmodel_v1/iac_v04_001_001/normal_mode/activate_normal_mode/normal_mode_fault_codes/iac_er_tmr2/Time Calculator/timer_calculation ==
  note: When 'reset_flag' is 1,
      |  'reset_value' is selected and
      | passed through the timer.
  note: 'init_value' provides the
      | initial value for the timer
  note: 'timer': cumulative
      | timer value
  note: 'Quantizer' switches the output
      |  to the appropriate resolution
      | based upon the top level
      |  dialog box selection.
  note: 'timer_calculation' takes the directional time increment 'delta_time'
      | and adds it to the previous timer value.  When the timer is reset,
      | all values are reset to 'reset_value'.
  reset_value : Inport
  reset_flag : Inport  Port=2
  delta_time : Inport  Port=3
  do_timer : TriggerPort  TriggerType=function-call  VariantControl=(inherit)
  Constant1 : Constant  Value=const_min
  Constant2 : Constant  Value=const_max
  Quantizer5 : Fcn  Expr=resolution*floor(u/resolution)
  Reset Switch : Switch  Threshold=0.5
  Sum : Sum  InputSameDT=on  SaturateOnIntegerOverflow=on  OutDataTypeStr=Inherit: Same as first input
  Terminator : Terminator
  Unit Delay : UnitDelay  InitialCondition=init_value  SampleTime=-1
  VAR SATURATION : Subsystem  mask(VARIABLE SATURATION){}
      mask help: This block will clip the input between the MIN and MAX values specified as inputs to the block. In addition a LIMIT_FLAG will be set to 1 if the input is currently being clipped.
      mask Display:
      | plot( [0.2 0.3 0.5 0.6], [0.2 0.2 0.8 0.8])
      | text(0.2, 0.05, 'min')
      | text(0.5, 0.95, 'max')
  lower bound = 0 : DeadZone  LowerValue=-inf  UpperValue=0.0
  timer : Outport  InitialOutput=0
  wires:
  Quantizer5/1 -> timer/1  "timer"
  VAR SATURATION/1(OUTPUT) -> Quantizer5/1, Unit Delay/1
  Sum/1 -> Reset Switch/3
  delta_time/1 -> Sum/1  "delta_time"
  reset_value/1 -> Reset Switch/1  "reset_value"
  reset_flag/1 -> Reset Switch/2  "reset_flag"
  Reset Switch/1 -> lower bound = 0/1
  Unit Delay/1 -> Sum/2  "previous  timer value"
  lower bound = 0/1 -> VAR SATURATION/2(INPUT)
  Constant1/1 -> VAR SATURATION/3(MIN)
  Constant2/1 -> VAR SATURATION/1(MAX)
  VAR SATURATION/2(LIMIT_FLAG) -> Terminator/1

== system mfordmodel_v1/iac_v04_001_001/normal_mode/activate_normal_mode/normal_mode_fault_codes/iac_mon_tmr/Time Calculator/delta_time ==
  note: timer14/TIMER/Time Calculator/delta_time
  note: Timer direction is represented by
      | the multiplier 'count_direction'
      | 'count_direction' can be either -1, 0, or 1.
  note: 'delta_time': the time interval
      | to be added to the timer for each cycle.
      | 'Gain' will adjust for second or millisecond timers.
  count_direction : Inport
  do_delta_time : TriggerPort  TriggerType=function-call  VariantControl=(inherit)
  Gain : Gain  Gain=unit_mul  SaturateOnIntegerOverflow=on  OutDataTypeStr=Inherit: Same as input  ParamDataTypeStr=Inherit: Same as input
  Product : Product  InputSameDT=on  RndMeth=Zero  SaturateOnIntegerOverflow=on  OutDataTypeStr=Inherit: Same as first input
  Realtime Digital Clock : DigitalClock  SampleTime=-1
  Sum : Sum  Inputs=+-  InputSameDT=on  SaturateOnIntegerOverflow=on  OutDataTypeStr=Inherit: Same as first input
  Unit Delay1 : UnitDelay  SampleTime=-1
  delta_time : Outport  InitialOutput=0
  wires:
  Realtime Digital Clock/1 -> Sum/1, Unit Delay1/1  "timer"
  Gain/1 -> Product/2
  Sum/1 -> Gain/1
  Unit Delay1/1 -> Sum/2
  Product/1 -> delta_time/1  "delta_time"
  count_direction/1 -> Product/1  "count_direction"

== system mfordmodel_v1/iac_v04_001_001/normal_mode/activate_normal_mode/normal_mode_fault_codes/iac_mon_tmr/Time Calculator/timer_calculation ==
  note: When 'reset_flag' is 1,
      |  'reset_value' is selected and
      | passed through the timer.
  note: 'init_value' provides the
      | initial value for the timer
  note: 'timer': cumulative
      | timer value
  note: 'Quantizer' switches the output
      |  to the appropriate resolution
      | based upon the top level
      |  dialog box selection.
  note: 'timer_calculation' takes the directional time increment 'delta_time'
      | and adds it to the previous timer value.  When the timer is reset,
      | all values are reset to 'reset_value'.
  reset_value : Inport
  reset_flag : Inport  Port=2
  delta_time : Inport  Port=3
  do_timer : TriggerPort  TriggerType=function-call  VariantControl=(inherit)
  Constant1 : Constant  Value=const_min
  Constant2 : Constant  Value=const_max
  Quantizer5 : Fcn  Expr=resolution*floor(u/resolution)
  Reset Switch : Switch  Threshold=0.5
  Sum : Sum  InputSameDT=on  SaturateOnIntegerOverflow=on  OutDataTypeStr=Inherit: Same as first input
  Terminator : Terminator
  Unit Delay : UnitDelay  InitialCondition=init_value  SampleTime=-1
  VAR SATURATION : Subsystem  mask(VARIABLE SATURATION){}
      mask help: This block will clip the input between the MIN and MAX values specified as inputs to the block. In addition a LIMIT_FLAG will be set to 1 if the input is currently being clipped.
      mask Display:
      | plot( [0.2 0.3 0.5 0.6], [0.2 0.2 0.8 0.8])
      | text(0.2, 0.05, 'min')
      | text(0.5, 0.95, 'max')
  lower bound = 0 : DeadZone  LowerValue=-inf  UpperValue=0.0
  timer : Outport  InitialOutput=0
  wires:
  Quantizer5/1 -> timer/1  "timer"
  VAR SATURATION/1(OUTPUT) -> Quantizer5/1, Unit Delay/1
  Sum/1 -> Reset Switch/3
  delta_time/1 -> Sum/1  "delta_time"
  reset_value/1 -> Reset Switch/1  "reset_value"
  reset_flag/1 -> Reset Switch/2  "reset_flag"
  Reset Switch/1 -> lower bound = 0/1
  Unit Delay/1 -> Sum/2  "previous  timer value"
  lower bound = 0/1 -> VAR SATURATION/2(INPUT)
  Constant1/1 -> VAR SATURATION/3(MIN)
  Constant2/1 -> VAR SATURATION/1(MAX)
  VAR SATURATION/2(LIMIT_FLAG) -> Terminator/1

== system mfordmodel_v1/iac_v04_001_001/normal_mode/iscflg_module/dashpot/TIMER/Time Calculator/delta_time ==
  note: timer14/TIMER/Time Calculator/delta_time
  note: Timer direction is represented by
      | the multiplier 'count_direction'
      | 'count_direction' can be either -1, 0, or 1.
  note: 'delta_time': the time interval
      | to be added to the timer for each cycle.
      | 'Gain' will adjust for second or millisecond timers.
  count_direction : Inport
  do_delta_time : TriggerPort  TriggerType=function-call  VariantControl=(inherit)
  Gain : Gain  Gain=unit_mul  SaturateOnIntegerOverflow=on  OutDataTypeStr=Inherit: Same as input  ParamDataTypeStr=Inherit: Same as input
  Product : Product  InputSameDT=on  RndMeth=Zero  SaturateOnIntegerOverflow=on  OutDataTypeStr=Inherit: Same as first input
  Realtime Digital Clock : DigitalClock  SampleTime=-1
  Sum : Sum  Inputs=+-  InputSameDT=on  SaturateOnIntegerOverflow=on  OutDataTypeStr=Inherit: Same as first input
  Unit Delay1 : UnitDelay  SampleTime=-1
  delta_time : Outport  InitialOutput=0
  wires:
  Realtime Digital Clock/1 -> Sum/1, Unit Delay1/1  "timer"
  Gain/1 -> Product/2
  Sum/1 -> Gain/1
  Unit Delay1/1 -> Sum/2
  Product/1 -> delta_time/1  "delta_time"
  count_direction/1 -> Product/1  "count_direction"

== system mfordmodel_v1/iac_v04_001_001/normal_mode/iscflg_module/dashpot/TIMER/Time Calculator/timer_calculation ==
  note: When 'reset_flag' is 1,
      |  'reset_value' is selected and
      | passed through the timer.
  note: 'init_value' provides the
      | initial value for the timer
  note: 'timer': cumulative
      | timer value
  note: 'Quantizer' switches the output
      |  to the appropriate resolution
      | based upon the top level
      |  dialog box selection.
  note: 'timer_calculation' takes the directional time increment 'delta_time'
      | and adds it to the previous timer value.  When the timer is reset,
      | all values are reset to 'reset_value'.
  reset_value : Inport
  reset_flag : Inport  Port=2
  delta_time : Inport  Port=3
  do_timer : TriggerPort  TriggerType=function-call  VariantControl=(inherit)
  Constant1 : Constant  Value=const_min
  Constant2 : Constant  Value=const_max
  Quantizer5 : Fcn  Expr=resolution*floor(u/resolution)
  Reset Switch : Switch  Threshold=0.5
  Sum : Sum  InputSameDT=on  SaturateOnIntegerOverflow=on  OutDataTypeStr=Inherit: Same as first input
  Terminator : Terminator
  Unit Delay : UnitDelay  InitialCondition=init_value  SampleTime=-1
  VAR SATURATION : Subsystem  mask(VARIABLE SATURATION){}
      mask help: This block will clip the input between the MIN and MAX values specified as inputs to the block. In addition a LIMIT_FLAG will be set to 1 if the input is currently being clipped.
      mask Display:
      | plot( [0.2 0.3 0.5 0.6], [0.2 0.2 0.8 0.8])
      | text(0.2, 0.05, 'min')
      | text(0.5, 0.95, 'max')
  lower bound = 0 : DeadZone  LowerValue=-inf  UpperValue=0.0
  timer : Outport  InitialOutput=0
  wires:
  Quantizer5/1 -> timer/1  "timer"
  VAR SATURATION/1(OUTPUT) -> Quantizer5/1, Unit Delay/1
  Sum/1 -> Reset Switch/3
  delta_time/1 -> Sum/1  "delta_time"
  reset_value/1 -> Reset Switch/1  "reset_value"
  reset_flag/1 -> Reset Switch/2  "reset_flag"
  Reset Switch/1 -> lower bound = 0/1
  Unit Delay/1 -> Sum/2  "previous  timer value"
  lower bound = 0/1 -> VAR SATURATION/2(INPUT)
  Constant1/1 -> VAR SATURATION/3(MIN)
  Constant2/1 -> VAR SATURATION/1(MAX)
  VAR SATURATION/2(LIMIT_FLAG) -> Terminator/1

== system mfordmodel_v1/iac_v04_001_001/normal_mode/iscflg_module/iscflg_modes/1/Time Calculator/delta_time ==
  note: timer14/TIMER/Time Calculator/delta_time
  note: Timer direction is represented by
      | the multiplier 'count_direction'
      | 'count_direction' can be either -1, 0, or 1.
  note: 'delta_time': the time interval
      | to be added to the timer for each cycle.
      | 'Gain' will adjust for second or millisecond timers.
  count_direction : Inport
  do_delta_time : TriggerPort  TriggerType=function-call  VariantControl=(inherit)
  Gain : Gain  Gain=unit_mul  SaturateOnIntegerOverflow=on  OutDataTypeStr=Inherit: Same as input  ParamDataTypeStr=Inherit: Same as input
  Product : Product  InputSameDT=on  RndMeth=Zero  SaturateOnIntegerOverflow=on  OutDataTypeStr=Inherit: Same as first input
  Realtime Digital Clock : DigitalClock  SampleTime=-1
  Sum : Sum  Inputs=+-  InputSameDT=on  SaturateOnIntegerOverflow=on  OutDataTypeStr=Inherit: Same as first input
  Unit Delay1 : UnitDelay  SampleTime=-1
  delta_time : Outport  InitialOutput=0
  wires:
  Realtime Digital Clock/1 -> Sum/1, Unit Delay1/1  "timer"
  Gain/1 -> Product/2
  Sum/1 -> Gain/1
  Unit Delay1/1 -> Sum/2
  Product/1 -> delta_time/1  "delta_time"
  count_direction/1 -> Product/1  "count_direction"

== system mfordmodel_v1/iac_v04_001_001/normal_mode/iscflg_module/iscflg_modes/1/Time Calculator/timer_calculation ==
  note: When 'reset_flag' is 1,
      |  'reset_value' is selected and
      | passed through the timer.
  note: 'init_value' provides the
      | initial value for the timer
  note: 'timer': cumulative
      | timer value
  note: 'Quantizer' switches the output
      |  to the appropriate resolution
      | based upon the top level
      |  dialog box selection.
  note: 'timer_calculation' takes the directional time increment 'delta_time'
      | and adds it to the previous timer value.  When the timer is reset,
      | all values are reset to 'reset_value'.
  reset_value : Inport
  reset_flag : Inport  Port=2
  delta_time : Inport  Port=3
  do_timer : TriggerPort  TriggerType=function-call  VariantControl=(inherit)
  Constant1 : Constant  Value=const_min
  Constant2 : Constant  Value=const_max
  Quantizer5 : Fcn  Expr=resolution*floor(u/resolution)
  Reset Switch : Switch  Threshold=0.5
  Sum : Sum  InputSameDT=on  SaturateOnIntegerOverflow=on  OutDataTypeStr=Inherit: Same as first input
  Terminator : Terminator
  Unit Delay : UnitDelay  InitialCondition=init_value  SampleTime=-1
  VAR SATURATION : Subsystem  mask(VARIABLE SATURATION){}
      mask help: This block will clip the input between the MIN and MAX values specified as inputs to the block. In addition a LIMIT_FLAG will be set to 1 if the input is currently being clipped.
      mask Display:
      | plot( [0.2 0.3 0.5 0.6], [0.2 0.2 0.8 0.8])
      | text(0.2, 0.05, 'min')
      | text(0.5, 0.95, 'max')
  lower bound = 0 : DeadZone  LowerValue=-inf  UpperValue=0.0
  timer : Outport  InitialOutput=0
  wires:
  Quantizer5/1 -> timer/1  "timer"
  VAR SATURATION/1(OUTPUT) -> Quantizer5/1, Unit Delay/1
  Sum/1 -> Reset Switch/3
  delta_time/1 -> Sum/1  "delta_time"
  reset_value/1 -> Reset Switch/1  "reset_value"
  reset_flag/1 -> Reset Switch/2  "reset_flag"
  Reset Switch/1 -> lower bound = 0/1
  Unit Delay/1 -> Sum/2  "previous  timer value"
  lower bound = 0/1 -> VAR SATURATION/2(INPUT)
  Constant1/1 -> VAR SATURATION/3(MIN)
  Constant2/1 -> VAR SATURATION/1(MAX)
  VAR SATURATION/2(LIMIT_FLAG) -> Terminator/1

== system mfordmodel_v1/iac_v04_001_001/normal_mode/iscflg_module/iscflg_modes/2/Time Calculator/delta_time ==
  note: timer14/TIMER/Time Calculator/delta_time
  note: Timer direction is represented by
      | the multiplier 'count_direction'
      | 'count_direction' can be either -1, 0, or 1.
  note: 'delta_time': the time interval
      | to be added to the timer for each cycle.
      | 'Gain' will adjust for second or millisecond timers.
  count_direction : Inport
  do_delta_time : TriggerPort  TriggerType=function-call  VariantControl=(inherit)
  Gain : Gain  Gain=unit_mul  SaturateOnIntegerOverflow=on  OutDataTypeStr=Inherit: Same as input  ParamDataTypeStr=Inherit: Same as input
  Product : Product  InputSameDT=on  RndMeth=Zero  SaturateOnIntegerOverflow=on  OutDataTypeStr=Inherit: Same as first input
  Realtime Digital Clock : DigitalClock  SampleTime=-1
  Sum : Sum  Inputs=+-  InputSameDT=on  SaturateOnIntegerOverflow=on  OutDataTypeStr=Inherit: Same as first input
  Unit Delay1 : UnitDelay  SampleTime=-1
  delta_time : Outport  InitialOutput=0
  wires:
  Realtime Digital Clock/1 -> Sum/1, Unit Delay1/1  "timer"
  Gain/1 -> Product/2
  Sum/1 -> Gain/1
  Unit Delay1/1 -> Sum/2
  Product/1 -> delta_time/1  "delta_time"
  count_direction/1 -> Product/1  "count_direction"

== system mfordmodel_v1/iac_v04_001_001/normal_mode/iscflg_module/iscflg_modes/2/Time Calculator/timer_calculation ==
  note: When 'reset_flag' is 1,
      |  'reset_value' is selected and
      | passed through the timer.
  note: 'init_value' provides the
      | initial value for the timer
  note: 'timer': cumulative
      | timer value
  note: 'Quantizer' switches the output
      |  to the appropriate resolution
      | based upon the top level
      |  dialog box selection.
  note: 'timer_calculation' takes the directional time increment 'delta_time'
      | and adds it to the previous timer value.  When the timer is reset,
      | all values are reset to 'reset_value'.
  reset_value : Inport
  reset_flag : Inport  Port=2
  delta_time : Inport  Port=3
  do_timer : TriggerPort  TriggerType=function-call  VariantControl=(inherit)
  Constant1 : Constant  Value=const_min
  Constant2 : Constant  Value=const_max
  Quantizer5 : Fcn  Expr=resolution*floor(u/resolution)
  Reset Switch : Switch  Threshold=0.5
  Sum : Sum  InputSameDT=on  SaturateOnIntegerOverflow=on  OutDataTypeStr=Inherit: Same as first input
  Terminator : Terminator
  Unit Delay : UnitDelay  InitialCondition=init_value  SampleTime=-1
  VAR SATURATION : Subsystem  mask(VARIABLE SATURATION){}
      mask help: This block will clip the input between the MIN and MAX values specified as inputs to the block. In addition a LIMIT_FLAG will be set to 1 if the input is currently being clipped.
      mask Display:
      | plot( [0.2 0.3 0.5 0.6], [0.2 0.2 0.8 0.8])
      | text(0.2, 0.05, 'min')
      | text(0.5, 0.95, 'max')
  lower bound = 0 : DeadZone  LowerValue=-inf  UpperValue=0.0
  timer : Outport  InitialOutput=0
  wires:
  Quantizer5/1 -> timer/1  "timer"
  VAR SATURATION/1(OUTPUT) -> Quantizer5/1, Unit Delay/1
  Sum/1 -> Reset Switch/3
  delta_time/1 -> Sum/1  "delta_time"
  reset_value/1 -> Reset Switch/1  "reset_value"
  reset_flag/1 -> Reset Switch/2  "reset_flag"
  Reset Switch/1 -> lower bound = 0/1
  Unit Delay/1 -> Sum/2  "previous  timer value"
  lower bound = 0/1 -> VAR SATURATION/2(INPUT)
  Constant1/1 -> VAR SATURATION/3(MIN)
  Constant2/1 -> VAR SATURATION/1(MAX)
  VAR SATURATION/2(LIMIT_FLAG) -> Terminator/1
